simulink model "vipconcentricity"  (R2015b)
settings: Solver=FixedStepDiscrete  StartTime=0.0  StopTime=inf  RelTol=1e-3
model workspace (MATLAB code in the model file):
  | NumPts=250;
undefined symbols (not defined in the file or in its folder): gray, Rec, SDTV, vipsimdelay
libraries: visiontextngfix x5, simulink x2, visionanalysis x2, visionsinks x2, visionstatistics x2, dspvision x1, vipmisc x1, visionconversions x1
settings Model: FPTRunName=Active  ExtModeAutoUpdateStatusClock=off  Creator=The MathWorks, Inc.  LastModifiedBy=The MathWorks, Inc.
settings DataIOCC: SaveFormat=Array  SaveOutput=off  SaveTime=off
settings OptimizationCC: ExpressionDepthLimit=2147483647  InitFltsAndDblsToZero=on
settings DebuggingCC: UnderspecifiedInitializationDetection=Classic  MergeDetectMultiDrivingBlocksExec=none  SignalResolutionControl=TryResolveAllWithWarning  SolverPrmCheckMsg=warning  InheritedTsInSrcMsg=none  MultiTaskDSMMsg=warning  MultiTaskCondExecSysMsg=none  FcnCallInpInsideContextMsg=UseLocalSettings  StateNameClashWarn=warning  StrictBusMsg=Warning
settings HardwareCC: ProdBitPerPointer=32  ProdLargestAtomicFloat=None  ProdIntDivRoundTo=Undefined  ProdEndianess=Unspecified  ProdWordSize=32  ProdHWDeviceType=32-bit Generic  TargetBitPerLong=64  TargetBitPerPointer=64  TargetLongLongMode=on  TargetIntDivRoundTo=Zero  TargetEndianess=LittleEndian  TargetWordSize=64  TargetHWDeviceType=Generic->MATLAB Host Computer  ProdEqTarget=off
settings SFSimCC: SimParseCustomCode=off
settings GRTTargetCC: TargetFcnLib=ansi_tfl_tmw_new.mat  GeneratePreprocessorConditionals=Disable all  CombineOutputUpdateFcns=off  GRTInterface=on
settings ConfigComp: CovModelRefEnable=Off

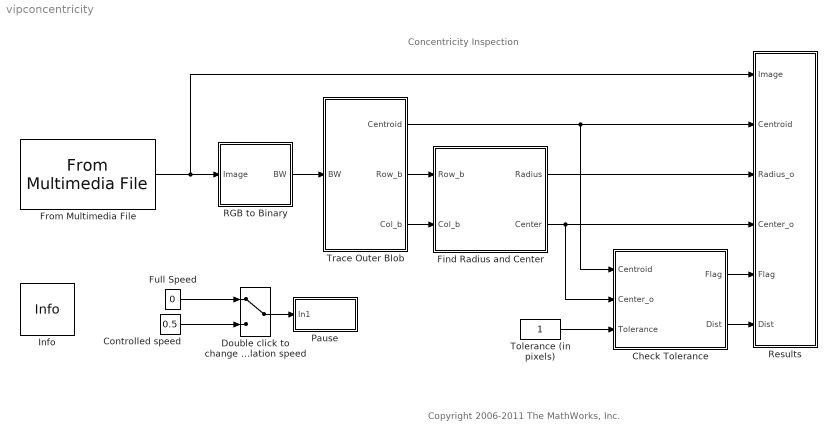
== system vipconcentricity ==
  note: Concentricity Inspection
  note: Copyright 2006-2011 The MathWorks, Inc.
  Check Tolerance : Subsystem
  Controlled speed : Constant  Value=0.5  VectorParams1D=off
  Double click to change the simulation speed : ManualSwitch
  Find Radius and Center : Subsystem
  From Multimedia File : dspvision/From Multimedia File  inputFilename=vipconcentricity.avi  loop=on  numPlays=inf  outputStreams=Video only  videoDataType=single  audioDataType=int16  inheritSampleTime=on  userDefinedSampleTime=1/15  noAudioOutput=off  isIntensityVideo=off  fourcc=RGB  colorVideoFormat=One multidimensional signal  outputEOF=off  dataOrg=Column-major  audioFrameSize=1024  computeAudioFrameSize=off  outSamplingMode=Frame based
  Full Speed : Constant  Value=0  VectorParams1D=off
  Info : vipmisc/Info  SystemSampleTime=-1
  Pause : Subsystem  TreatAsAtomicUnit=on  SimViewingDevice=on
      mask Display: disp('Pause');
  RGB to Binary : Subsystem
  Results : Subsystem
  Tolerance (in pixels) : Constant  VectorParams1D=off  OutDataTypeStr=int32
  Trace Outer Blob : Subsystem
  wires:
  From Multimedia File/1 -> RGB to Binary/1(Image), Results/1(Image)
  Trace Outer Blob/2(Row_b) -> Find Radius and Center/1(Row_b)
  Trace Outer Blob/3(Col_b) -> Find Radius and Center/2(Col_b)
  RGB to Binary/1(BW) -> Trace Outer Blob/1(BW)
  Trace Outer Blob/1(Centroid) -> Results/2(Centroid), Check Tolerance/1(Centroid)
  Check Tolerance/1(Flag) -> Results/5(Flag)
  Tolerance (in pixels)/1 -> Check Tolerance/3(Tolerance)
  Check Tolerance/2(Dist) -> Results/6(Dist)
  Double click to change the simulation speed/1 -> Pause/1(In1)
  Full Speed/1 -> Double click to change the simulation speed/1
  Controlled speed/1 -> Double click to change the simulation speed/2
  Find Radius and Center/2(Center) -> Results/4(Center_o), Check Tolerance/2(Center_o)
  Find Radius and Center/1(Radius) -> Results/3(Radius_o)

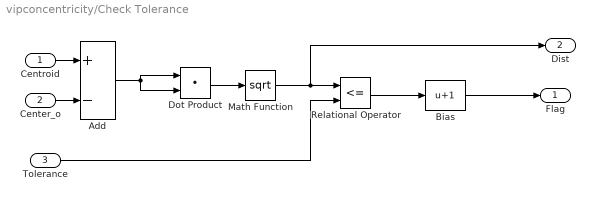
== system vipconcentricity/Check Tolerance ==
  Centroid : Inport
  Center_o : Inport  Port=2
  Tolerance : Inport  Port=3
  Add : Sum  Inputs=+-
  Bias : Bias  Bias=1
  Dot Product : DotProduct  InputSameDT=on  OutDataTypeStr=Inherit: Inherit via internal rule
  Math Function : Math  Operator=sqrt  SaturateOnIntegerOverflow=on
  Relational Operator : RelationalOperator  Operator=<=  OutDataTypeStr=fixdt(1,32)
  Flag : Outport
  Dist : Outport  Port=2
  wires:
  Add/1 -> Dot Product/1, Dot Product/2
  Dot Product/1 -> Math Function/1
  Relational Operator/1 -> Bias/1
  Centroid/1 -> Add/1
  Center_o/1 -> Add/2
  Tolerance/1 -> Relational Operator/2
  Math Function/1 -> Relational Operator/1, Dist/1
  Bias/1 -> Flag/1

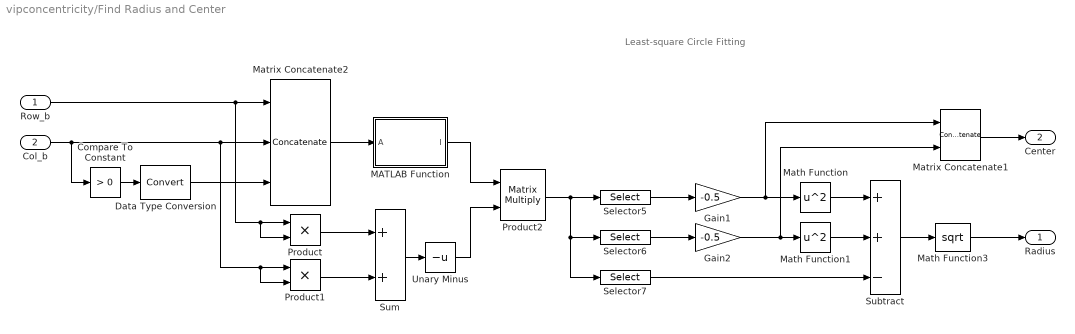
== system vipconcentricity/Find Radius and Center ==
  note: Least-square Circle Fitting
  Row_b : Inport
  Col_b : Inport  Port=2
  Compare To Constant : simulink/Logic and Bit Operations/Compare To Constant  relop=>  const=0  OutDataTypeStr=uint8
  Data Type Conversion : DataTypeConversion
  Gain1 : Gain  Gain=-0.5
  Gain2 : Gain  Gain=-0.5
  MATLAB Function : MATLAB Function  TreatAsAtomicUnit=on
  Math Function : Math  Operator=square  SaturateOnIntegerOverflow=on
  Math Function1 : Math  Operator=square  SaturateOnIntegerOverflow=on
  Math Function3 : Math  Operator=sqrt  SaturateOnIntegerOverflow=on
  Matrix Concatenate1 : Concatenate  Mode=Multidimensional array
  Matrix Concatenate2 : Concatenate  NumInputs=3  Mode=Multidimensional array  ConcatenateDimension=2
  Product : Product  RndMeth=Zero
  Product1 : Product  RndMeth=Zero
  Product2 : Product  Multiplication=Matrix(*)  RndMeth=Zero
  Selector5 : Selector  InputPortWidth=3  IndexOptions=Index vector (dialog)  Indices=(1)  OutputSizes=1
  Selector6 : Selector  InputPortWidth=3  IndexOptions=Index vector (dialog)  Indices=(2)  OutputSizes=1
  Selector7 : Selector  InputPortWidth=3  IndexOptions=Index vector (dialog)  Indices=(3)  OutputSizes=1
  Subtract : Sum  Inputs=++-
  Sum : Sum
  Unary Minus : UnaryMinus
  Radius : Outport
  Center : Outport  Port=2
  wires:
  Row_b/1 -> Product/1, Product/2, Matrix Concatenate2/1
  Col_b/1 -> Compare To Constant/1, Product1/1, Product1/2, Matrix Concatenate2/2
  Product/1 -> Sum/1
  Product1/1 -> Sum/2
  Product2/1 -> Selector5/1, Selector6/1, Selector7/1
  Matrix Concatenate2/1 -> MATLAB Function/1(A)
  Sum/1 -> Unary Minus/1
  MATLAB Function/1(I) -> Product2/1
  Unary Minus/1 -> Product2/2
  Selector6/1 -> Gain2/1
  Selector5/1 -> Gain1/1
  Gain1/1 -> Math Function/1, Matrix Concatenate1/1
  Gain2/1 -> Math Function1/1, Matrix Concatenate1/2
  Math Function1/1 -> Subtract/2
  Math Function/1 -> Subtract/1
  Selector7/1 -> Subtract/3
  Subtract/1 -> Math Function3/1
  Matrix Concatenate1/1 -> Center/1
  Math Function3/1 -> Radius/1
  Compare To Constant/1 -> Data Type Conversion/1
  Data Type Conversion/1 -> Matrix Concatenate2/3

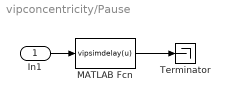
== system vipconcentricity/Pause ==
  In1 : Inport
  MATLAB Fcn : MATLABFcn  MATLABFcn=vipsimdelay(u)
  Terminator : Terminator
  wires:
  In1/1 -> MATLAB Fcn/1
  MATLAB Fcn/1 -> Terminator/1

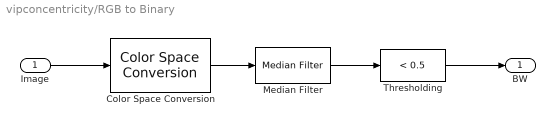
== system vipconcentricity/RGB to Binary ==
  Image : Inport
  Color Space Conversion : visionconversions/Color Space  Conversion  conversion=Obsolete  conversionActive=R'G'B' to intensity  wp_str=D65  rec=Rec. 601 (SDTV)  sys=1125/60/2:1  imagePorts=One multidimensional signal
  Median Filter : visionanalysis/Median Filter  nghbood=[3 3]  outSize=Same as input port I  padType=Replicate  padSrc=Specify via dialog  padVal=0  roundingMode=Floor  overflowMode=off
  Thresholding : simulink/Logic and Bit Operations/Compare To Constant  relop=<  const=0.5  OutDataTypeStr=boolean  ZeroCross=off
  BW : Outport
  wires:
  Median Filter/1 -> Thresholding/1
  Image/1 -> Color Space Conversion/1
  Thresholding/1 -> BW/1
  Color Space Conversion/1 -> Median Filter/1

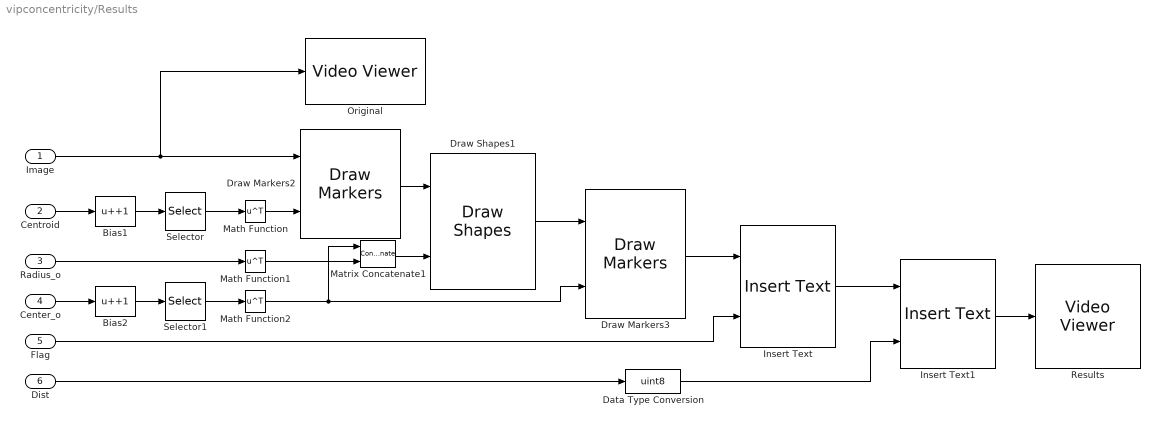
== system vipconcentricity/Results ==
  Image : Inport
  Centroid : Inport  Port=2
  Radius_o : Inport  Port=3
  Center_o : Inport  Port=4
  Flag : Inport  Port=5
  Dist : Inport  Port=6
  Bias1 : Bias  Bias=+1
  Bias2 : Bias  Bias=+1
  Data Type Conversion : DataTypeConversion  OutDataTypeStr=uint8  SaturateOnIntegerOverflow=on  RndMeth=Zero
  Draw Markers2 : visiontextngfix/Draw Markers  shape=Plus  size=3  fill=off  fillClrSource=Specify via dialog  display=User-specified value  intensity=155  color=[255 0 0]  opacity=1  viewport=Entire image  antialiasing=off  inType=Obsolete  imagePorts=One multidimensional signal  prodOutputMode=Binary point scaling  prodOutputWordLength=32  prodOutputFracLength=14  memoryMode=Specify word length  memoryWordLength=16  memoryFracLength=15  roundingMode=Floor  overflowMode=off
  Draw Markers3 : visiontextngfix/Draw Markers  shape=Star  size=3  fill=off  fillClrSource=Specify via dialog  display=User-specified value  intensity=155  color=[0 255 0]  opacity=1  viewport=Entire image  antialiasing=off  inType=Obsolete  imagePorts=One multidimensional signal  prodOutputMode=Binary point scaling  prodOutputWordLength=32  prodOutputFracLength=14  memoryMode=Specify word length  memoryWordLength=16  memoryFracLength=15  roundingMode=Floor  overflowMode=off
  Draw Shapes1 : visiontextngfix/Draw Shapes  shape=Circles  fill=off  lineWidth=1  fillClrSource=Specify via dialog  display=User-specified value  intensity=200  color=[0 1 1]  opacity=0.6  viewport=Entire image  antialiasing=off  inType=Obsolete  imagePorts=One multidimensional signal  prodOutputMode=Binary point scaling  prodOutputWordLength=32  prodOutputFracLength=14  memoryMode=Specify word length  memoryWordLength=16  memoryFracLength=15  roundingMode=Floor  overflowMode=off
  Insert Text : visiontextngfix/Insert Text  inputType=Obsolete  theText="{'Concentricity: Bad  ','Concentricity: Good'}"  getTextLocFrom=Specify via dialog  textLoc=[1 1]  getTextColorFrom=Specify via dialog  textColor=[0 0 0]  getTextIntensityFrom=Specify via dialog  textIntensity=0  getTextOpacityFrom=Specify via dialog  textOpacity=1.0  dummyVar2=0  dummyVar3=0  dummyVar4=0  imagePorts=One multidimensional signal  isInputTransposed=off  fontFace=LucidaBrightRegular  dummyVar1=0  blockFontSize=14  antiAliased=on
  Insert Text1 : visiontextngfix/Insert Text  inputType=Obsolete  theText='Distance in pixels: %2d '  getTextLocFrom=Specify via dialog  textLoc=[1 21]  getTextColorFrom=Specify via dialog  textColor=[0 0 0]  getTextIntensityFrom=Specify via dialog  textIntensity=0  getTextOpacityFrom=Specify via dialog  textOpacity=1.0  dummyVar2=0  dummyVar3=0  dummyVar4=0  imagePorts=One multidimensional signal  isInputTransposed=off  fontFace=LucidaBrightRegular  dummyVar1=0  blockFontSize=14  antiAliased=on
  Math Function : Math  Operator=transpose  SaturateOnIntegerOverflow=on
  Math Function1 : Math  Operator=transpose  SaturateOnIntegerOverflow=on
  Math Function2 : Math  Operator=transpose  SaturateOnIntegerOverflow=on
  Matrix Concatenate1 : Concatenate  Mode=Multidimensional array  ConcatenateDimension=2
  Original : visionsinks/Video Viewer  inputType=Obsolete7b  imagePorts=One multidimensional signal  useColorMap=off  colormapValue=gray(256)  specRange=off  minInputVal=0  maxInputVal=255  FigPos=[175 379 220 250]  AxisZoom=on  trueSizedOnce=on  OpenAtMdlStart=on  DefaultConfigurationName=vipscopes.VideoViewerScopeCfg
  Results : visionsinks/Video Viewer  inputType=Obsolete7b  imagePorts=One multidimensional signal  useColorMap=off  colormapValue=gray(256)  specRange=off  minInputVal=0  maxInputVal=255  FigPos=[413 381 238 252]  AxisZoom=on  trueSizedOnce=on  OpenAtMdlStart=on  DefaultConfigurationName=vipscopes.VideoViewerScopeCfg
  Selector : Selector  NumberOfDimensions=2  InputPortWidth=3  IndexOptions=Index vector (dialog),Select all  Indices=[2 1],[2 1]  OutputSizes=1,1
  Selector1 : Selector  NumberOfDimensions=2  InputPortWidth=3  IndexOptions=Index vector (dialog),Select all  Indices=[2 1],[2 1]  OutputSizes=1,1
  wires:
  Draw Markers2/1 -> Draw Shapes1/1
  Draw Shapes1/1 -> Draw Markers3/1
  Draw Markers3/1 -> Insert Text/1
  Image/1 -> Draw Markers2/1, Original/1
  Flag/1 -> Insert Text/2
  Insert Text/1 -> Insert Text1/1
  Dist/1 -> Data Type Conversion/1
  Data Type Conversion/1 -> Insert Text1/2
  Radius_o/1 -> Math Function1/1
  Matrix Concatenate1/1 -> Draw Shapes1/2
  Insert Text1/1 -> Results/1
  Centroid/1 -> Bias1/1
  Selector/1 -> Math Function/1
  Math Function/1 -> Draw Markers2/2
  Center_o/1 -> Bias2/1
  Selector1/1 -> Math Function2/1
  Math Function2/1 -> Matrix Concatenate1/1, Draw Markers3/2
  Math Function1/1 -> Matrix Concatenate1/2
  Bias1/1 -> Selector/1
  Bias2/1 -> Selector1/1

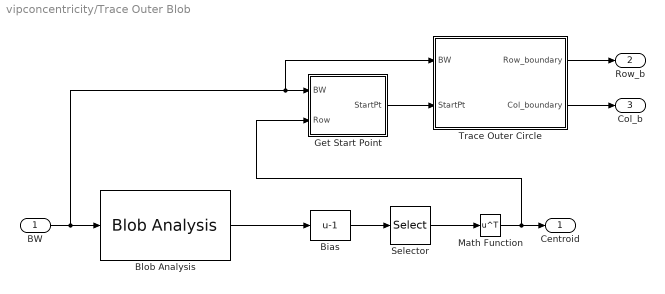
== system vipconcentricity/Trace Outer Blob ==
  BW : Inport
  Bias : Bias  Bias=-1
  Blob Analysis : visionstatistics/Blob Analysis  Tag=vipblks_row_conv  area=off  centroid=on  bBox=off  majorAxis=off  minorAxis=off  angle=off  eccentricity=off  equivDiameterSq=off  extent=off  perimeter=off  maxBlobs=1  warnIfNumBlobsExceeded=off  isCount=off  useMinArea=off  minArea=0  useMaxArea=off  maxArea=inf  excludeBorderBlob=off  outDT=single  isOutVarDim=off  isFill=on  fillValues=-1  conn=8  isLabel=off  outputMode=Binary point scaling  outputWordLength=32  outputFracLength=16  firstCoeffMode=Binary point scaling  firstCoeffWordLength=16  firstCoeffFracLength=14  secondCoeffMode=Binary point scaling  secondCoeffWordLength=32  secondCoeffFracLength=16  accumMode=Binary point scaling  accumWordLength=32  accumFracLength=0  prodOutputMode=Binary point scaling  prodOutputWordLength=32  prodOutputFracLength=16  roundingMode=Floor  overflowMode=off
  Get Start Point : Subsystem
  Math Function : Math  Operator=transpose  SaturateOnIntegerOverflow=on
  Selector : Selector  NumberOfDimensions=2  InputPortWidth=3  IndexOptions=Select all,Index vector (dialog)  Indices=[1 3],[2 1]  OutputSizes=1,1
  Trace Outer Circle : Subsystem
  Centroid : Outport
  Row_b : Outport  Port=2
  Col_b : Outport  Port=3
  wires:
  BW/1 -> Blob Analysis/1, Get Start Point/1(BW), Trace Outer Circle/1(BW)
  Get Start Point/1(StartPt) -> Trace Outer Circle/2(StartPt)
  Blob Analysis/1 -> Bias/1
  Bias/1 -> Selector/1
  Selector/1 -> Math Function/1
  Math Function/1 -> Get Start Point/2(Row), Centroid/1
  Trace Outer Circle/1(Row_boundary) -> Row_b/1
  Trace Outer Circle/2(Col_boundary) -> Col_b/1

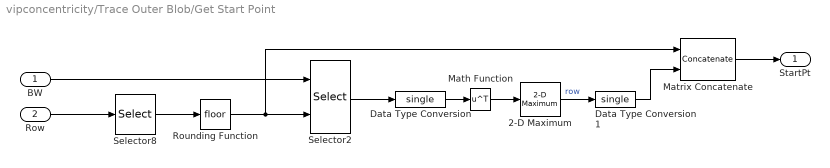
== system vipconcentricity/Trace Outer Blob/Get Start Point ==
  BW : Inport
  Row : Inport  Port=2
  2-D Maximum : visionstatistics/2-D Maximum  fcn=Index  reset=None  indexBase=One  operateOver=Each column  Dimension=1  colComp=off  operation=maximum  roiEnable=off  roiType=Rectangles  roiPortion=Entire ROI  roiOutput=Individual statistics for each ROI  roiFlag=off  accumDataTypeStr=Inherit: Same as product output  accumLastDataTypeStr=Inherit: Same as product output  roundingMode=Floor  overflowMode=off
  Data Type Conversion : DataTypeConversion  OutDataTypeStr=single  SaturateOnIntegerOverflow=on  RndMeth=Zero
  Data Type Conversion1 : DataTypeConversion  OutDataTypeStr=single  SaturateOnIntegerOverflow=on  RndMeth=Zero
  Math Function : Math  Operator=transpose  SaturateOnIntegerOverflow=on
  Matrix Concatenate : Concatenate  Mode=Multidimensional array
  Rounding Function : Rounding
  Selector2 : Selector  NumberOfDimensions=2  InputPortWidth=2  IndexOptions=Index vector (port),Select all  Indices=(-1),(-1)  OutputSizes=1
  Selector8 : Selector  InputPortWidth=2  IndexOptions=Index vector (dialog)  Indices=(1)  OutputSizes=1
  StartPt : Outport
  wires:
  Matrix Concatenate/1 -> StartPt/1
  Selector8/1 -> Rounding Function/1
  Selector2/1 -> Data Type Conversion/1
  Data Type Conversion1/1 -> Matrix Concatenate/2
  Data Type Conversion/1 -> Math Function/1
  2-D Maximum/1 -> Data Type Conversion1/1  "row"
  BW/1 -> Selector2/1
  Row/1 -> Selector8/1
  Rounding Function/1 -> Matrix Concatenate/1, Selector2/2
  Math Function/1 -> 2-D Maximum/1

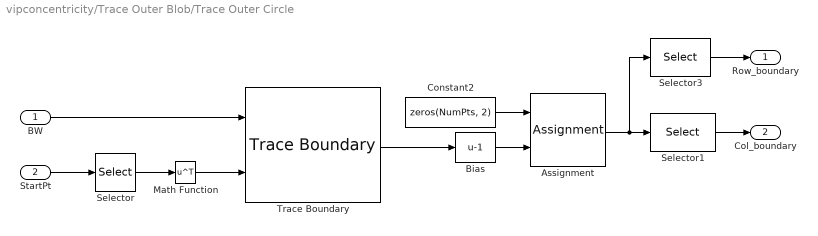
== system vipconcentricity/Trace Outer Blob/Trace Outer Circle ==
  BW : Inport
  StartPt : Inport  Port=2
  Assignment : Assignment  NumberOfDimensions=2  IndexOptions=Starting index (dialog),Assign all  Indices=1,1  OutputSizes=NumPts,2
  Bias : Bias  Bias=-1
  Constant2 : Constant  Value=zeros(NumPts, 2)  OutDataTypeStr=single
  Math Function : Math  Operator=transpose  SaturateOnIntegerOverflow=on
  Selector : Selector  InputPortWidth=2  IndexOptions=Index vector (dialog)  Indices=[2 1]  OutputSizes=1
  Selector1 : Selector  NumberOfDimensions=2  InputPortWidth=2*NumPts  IndexOptions=Select all,Index vector (dialog)  Indices=(2:2:(2*NumPts)),1  OutputSizes=1,1
  Selector3 : Selector  NumberOfDimensions=2  InputPortWidth=2*NumPts  IndexOptions=Select all,Index vector (dialog)  Indices=(2:2:(2*NumPts)),2  OutputSizes=1,1
  Trace Boundary : visionanalysis/Trace Boundary  conn=8  searchDir4=North  searchDir8=North  traceDir=Clockwise  maxNumPix=NumPts  outputNum=off  fillChoices=None  fillVal=[0 0]
  Row_boundary : Outport
  Col_boundary : Outport  Port=2
  wires:
  BW/1 -> Trace Boundary/1
  StartPt/1 -> Selector/1
  Selector/1 -> Math Function/1
  Assignment/1 -> Selector1/1, Selector3/1
  Selector3/1 -> Row_boundary/1
  Selector1/1 -> Col_boundary/1
  Constant2/1 -> Assignment/1
  Trace Boundary/1 -> Bias/1
  Math Function/1 -> Trace Boundary/2
  Bias/1 -> Assignment/2

== matlab function vipconcentricity/Find Radius and Center/MATLAB Function ==
  data: A input; I output
function I = pinv(A)
%#codegen

I = pinv(A);
